simulink model "extractLocal_simfcn"  (R2024b)
settings: Solver=FixedStepAuto  StartTime=0.0  StopTime=10.0  RelTol=1e-3
InitFcn:
  | extractLocalMapSetup
undefined symbols (not defined in the file): tuneableTEBParams, worldGridLoc, worldMat, worldRes
libraries: roshelperlib x1
settings Model: Creator=cstabile  LastModifiedBy=jbrault
settings SolverCC: DateTimeAtSimulationTimeZero=[]

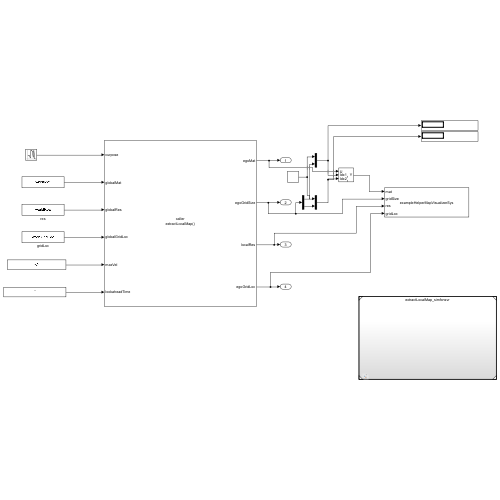
[thumbnail: Simulink's stored preview of the top-level diagram]
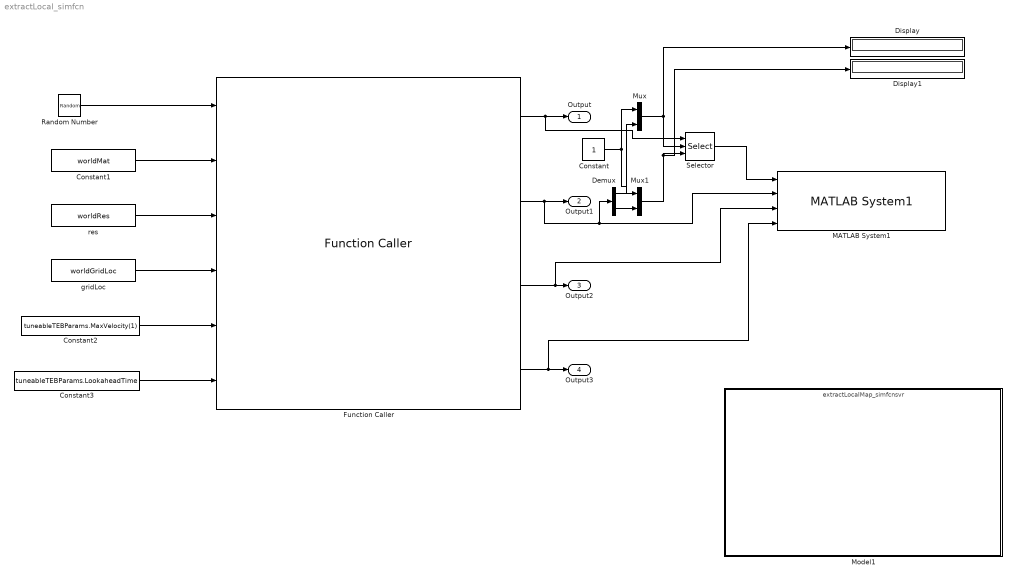
== system extractLocal_simfcn ==
  Constant : Constant
  Constant1 : Constant  Value=worldMat
  Constant2 : Constant  Value=tuneableTEBParams.MaxVelocity(1)
  Constant3 : Constant  Value=tuneableTEBParams.LookaheadTime
  Demux : Demux  Outputs=2
  Display : Display
  Display1 : Display
  Function Caller : FunctionCaller  FunctionPrototype=[egoMat,egoGridSize,localRes,egoGridLoc] = extractLocalMap(curpose,globalMat,globalRes,globalGridLoc,maxVel,lookaheadTime)  InputArgumentSpecifications=<Enter example>  OutputArgumentSpecifications=<Enter example>
  MATLAB System1 : roshelperlib/MATLAB System1  MapType=SDF  IsEgo=off  DisplayVisual=on  SimulateUsing=Interpreted execution
  Model1 : ModelReference  ModelNameDialog=extractLocalMap_simfcnsvr.slx  SimulationMode=Normal  ScheduleRates=on  ModelReferenceVersion=2.0
  Mux : Mux  Inputs=2
  Mux1 : Mux  Inputs=2
  Random Number : RandomNumber  Mean=[500 500 0]  Variance=[100 100 0]
  Selector : Selector  NumberOfDimensions=2  InputPortWidth=3  IndexOptions=Starting and ending indices (port),Starting and ending indices (port)  Indices=[1 3],1  OutputSizes=1,1
  gridLoc : Constant  Value=worldGridLoc  VectorParams1D=off
  res : Constant  Value=worldRes
  Output : Outport
  Output1 : Outport  Port=2
  Output2 : Outport  Port=3
  Output3 : Outport  Port=4
  wires:
  Random Number/1 -> Function Caller/1
  Constant1/1 -> Function Caller/2
  res/1 -> Function Caller/3
  gridLoc/1 -> Function Caller/4
  Function Caller/1 -> Selector/1, Output/1
  Constant2/1 -> Function Caller/5
  Function Caller/3 -> MATLAB System1/3, Output2/1
  Constant3/1 -> Function Caller/6
  Function Caller/2 -> MATLAB System1/2, Demux/1, Output1/1
  Function Caller/4 -> MATLAB System1/4, Output3/1
  Constant/1 -> Mux1/1, Mux/1
  Demux/1 -> Mux/2
  Demux/2 -> Mux1/2
  Mux1/1 -> Display1/1, Selector/3
  Mux/1 -> Display/1, Selector/2
  Selector/1 -> MATLAB System1/1
